simulink model "output"  (R2024b)
settings: Solver=FixedStepAuto  StartTime=0.0  StopTime=inf  RelTol=1e-3  EnableMultiTasking=on
libraries: stm32f4xxblockslib x6, spsACVoltageSourceLib x1, ee_lib x1
settings Model: STM32="{\"AnalogInput\":[{\"ID\":\"untitled:1\"},{\"ID\":\"kuay:1\"},{\"ID\":\"kuay:9\"},{\"ID\":\"kuay:13\"},{\"ID\":\"kuay:16\"},{\"ID\":\"output:16\"},{\"ID\":\"output:13\"},{\"ID\":\"output:9\"},{\"ID\":\"output:1\"}],\"DigitalPortWrite\":[{\"ID\":\"kuay:5\"},{\"ID\":\"output:5\"}],\"DigitalPortRead\":[{\"ID\":\"kuay:6\"},{\"ID\":\"output:6\"}]}"  Creator=Sasish  LastModifiedBy=Sasish
settings OptimizationCC: DefaultParameterBehavior=Inlined  EnhancedBackFolding=on  PassReuseOutputArgsAs=Individual arguments  ZeroExternalMemoryAtStartup=off  ZeroInternalMemoryAtStartup=off  MaxStackSize=512  OptimizeBlockOrder=speed  DifferentSizesBufferReuse=on  OptimizationCustomize=off  EfficientTunableParamExpr=on
settings DebuggingCC: ParameterTunabilityLossMsg=error
settings HardwareCC: ProdBitPerPointer=32  ProdBitPerSizeT=32  ProdBitPerPtrDiffT=32  ProdLargestAtomicInteger=Long  ProdLargestAtomicFloat=Double  ProdWordSize=32  ProdLongLongMode=on  ProdHWDeviceType=ARM Compatible->ARM Cortex-M
settings SFSimCC: MATLABDynamicMemAlloc=off
settings RTWCC: Description=Embedded Coder  SystemTargetFile=ert.tlc  HardwareBoard=STM32G4xx Based  TemplateMakefile=ert_default_tmf  Toolchain=GNU Tools for ARM Embedded Processors
settings CodeAppCC: ForceParamTrailComments=on  IgnoreCustomStorageClasses=off  OperatorAnnotations=on  SimulinkDataObjDesc=on  SFDataObjDesc=on  InsertBlockDesc=on
settings ERTTargetCC: TargetLangStandard=C99 (ISO)  CodeReplacementLibrary=ARM Cortex-M  ExtModeTransport=3  ExtModeStaticAlloc=on  ExtModeStaticAllocSize=2048  ExtModeMexFile=ext_xcp  ExtModeIntrfLevel=Level2 - Open

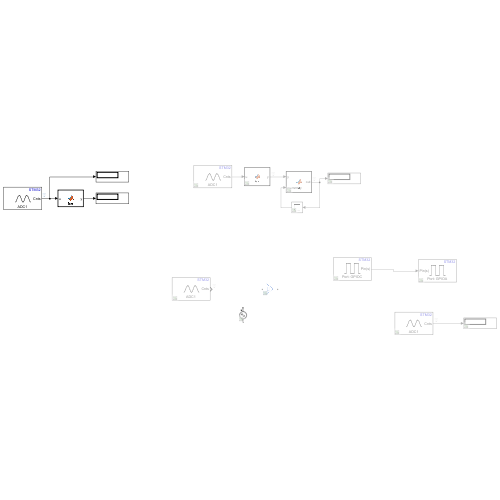
[thumbnail: Simulink's stored preview of the top-level diagram]
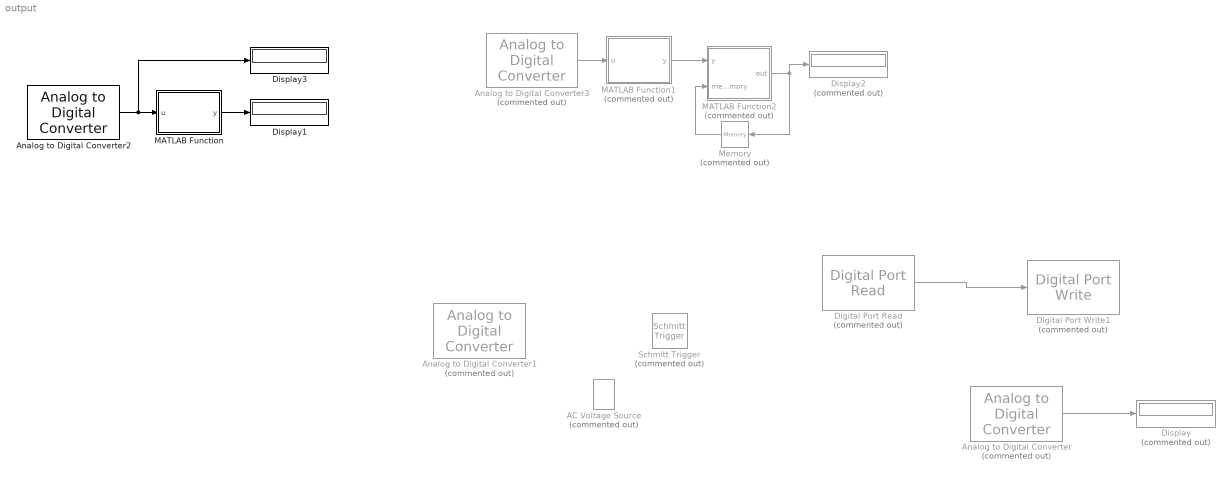
== system output ==
  AC Voltage Source : spsACVoltageSourceLib/AC Voltage Source  Commented=on  Amplitude=100  Phase=0  Frequency=60  SampleTime=0  Measurements=None  BusType=swing  Pref=10e3  Qref=0  Qmin=-inf  Qmax=+inf
  Analog to Digital Converter : stm32f4xxblockslib/Analog to Digital Converter  Commented=on  ADCModule=ADC1  ConversionGroup=Regular  TriggerMode=Trigger and read  NumberOfConversions=1  EnableBufferConv=off  BufferLength=1  OutputStatus=off  SampleTime=-1  EnableSimPort=off  hoistedMaskSrc=ECSoC/ECSimCodegen/Analog to Digital Converter
  Analog to Digital Converter1 : stm32f4xxblockslib/Analog to Digital Converter  Commented=on  ADCModule=ADC1  ConversionGroup=Regular  TriggerMode=Trigger and read  NumberOfConversions=1  EnableBufferConv=off  BufferLength=1  OutputStatus=off  SampleTime=-1  EnableSimPort=off  hoistedMaskSrc=ECSoC/ECSimCodegen/Analog to Digital Converter
  Analog to Digital Converter2 : stm32f4xxblockslib/Analog to Digital Converter  ADCModule=ADC1  ConversionGroup=Regular  TriggerMode=Trigger and read  NumberOfConversions=1  EnableBufferConv=off  BufferLength=1  OutputStatus=off  SampleTime=-1  EnableSimPort=off  hoistedMaskSrc=ECSoC/ECSimCodegen/Analog to Digital Converter
  Analog to Digital Converter3 : stm32f4xxblockslib/Analog to Digital Converter  Commented=on  ADCModule=ADC1  ConversionGroup=Regular  TriggerMode=Trigger and read  NumberOfConversions=1  EnableBufferConv=off  BufferLength=1  OutputStatus=off  SampleTime=-1  EnableSimPort=off  hoistedMaskSrc=ECSoC/ECSimCodegen/Analog to Digital Converter
  Digital Port Read : stm32f4xxblockslib/Digital Port Read  Commented=on  PortName=GPIOC  PinNumber=[13]  ReadOperation=on  IOAsArray=on  SampleTime=-1  EnableSimPort=off  hoistedMaskSrc=ECSoC/ECSimCodegen/Digital Port Read
      settings: LibrarySourceBlock=stm32g4xxblockslib/Digital Port Read
  Digital Port Write1 : stm32f4xxblockslib/Digital Port Write  Commented=on  PortName=GPIOA  PinNumber=[5]  ReadOperation=off  IOAsArray=on  EnableSimPort=off  hoistedMaskSrc=ECSoC/ECSimCodegen/Digital Port Write
      settings: LibrarySourceBlock=stm32g4xxblockslib/Digital Port Write
  Display : Display  Commented=on
  Display1 : Display
  Display2 : Display  Commented=on
  Display3 : Display
  MATLAB Function : MATLAB Function  TreatAsAtomicUnit=on
  MATLAB Function1 : MATLAB Function  Commented=on  TreatAsAtomicUnit=on
  MATLAB Function2 : MATLAB Function  Commented=on  TreatAsAtomicUnit=on
  Memory : Memory  Commented=on
  Schmitt Trigger : ee_lib/Integrated Circuits/Logic/Schmitt Trigger  Commented=on  V_IL=2 V  V_IH=3 V  C_IN=5 pF  output_type=ee.enum.ic.outputType.linear  V_OL=0 V  V_OH=5 V  V_CC=5 V  V_meas=5 V  R_OUT=25 Ohm  R_OH=[25, 250] Ohm  I_OH=63 mA  R_OL=[30, 800] Ohm  I_OL=-45 mA  Delay=25 ns  Ron=5 Ohm  Vf=0.6 V  output_state=ee.enum.ic.initialState.low
      settings: InternalSimscapePortConfiguration="{\"Bottom\":[],\"Left\":[{\"id\":\"A\",\"label\":\"\",\"type\":\"foundation.electrical.electrical\"}],\"Right\":[{\"id\":\"J\",\"label\":\"\",\"type\":\"foundation.electrical.electrical\"}],\"Top\":[]}"
  wires:
  Analog to Digital Converter/1 -> Display/1
  Digital Port Read/1 -> Digital Port Write1/1
  Analog to Digital Converter2/1 -> Display3/1, MATLAB Function/1(u)
  MATLAB Function/1(y) -> Display1/1
  Analog to Digital Converter3/1 -> MATLAB Function1/1(u)
  MATLAB Function1/1(y) -> MATLAB Function2/1(y)
  MATLAB Function2/1(out) -> Memory/1, Display2/1
  Memory/1 -> MATLAB Function2/2(memmory)

== matlab function output/MATLAB Function1 ==
  data: u input; y output
function y = fcn(u)
in_min= 0;
out_min=0;
out_max=1;
in_max=4095;
y= double(u - in_min) * (out_max - out_min) / (in_max - in_min) + out_min;

== matlab function output/MATLAB Function ==
  data: u input; y output
function y = fcn(u)
in_min= 0;
out_min=0;
out_max=3.3;
in_max=4095;
y= double(u - in_min) * (out_max - out_min) / (in_max - in_min) + out_min;

== matlab function output/MATLAB Function2 ==
  data: y input; memmory input; out output
function out = fcn(y,memmory)
if y >= 0.7
    out=1;
elseif y <= 0.3
    out=0;
else
    out = memmory;
end
